simulink model "seesaw"  (Simulink 4.00)
settings: Solver=ode45  StartTime=0.0  StopTime=40  RelTol=1e-3
settings Model: Creator=tjanas  LastModifiedBy=tjanas  ExtModeAutoUpdateStatusClock=off  BooleanDataType=on

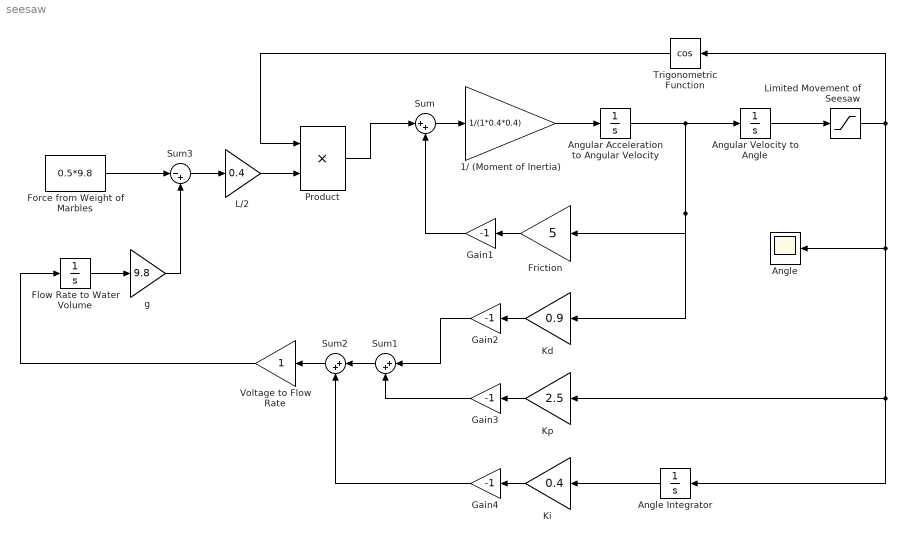
== system seesaw ==
  1/ (Moment of Inertia) : Gain  Gain=1/(1*0.4*0.4)  Multiplication=Element-wise(K.*u)  SaturateOnIntegerOverflow=on
  Angle : Scope
      settings: TimeRange=auto  YMin=-5  YMax=5  SaveToWorkspace=off  SaveName=ScopeData  LimitDataPoints=on  MaxDataPoints=5000
  Angle Integrator : Integrator  Orientation=left  ExternalReset=none  InitialConditionSource=internal  InitialCondition=1  LimitOutput=off  UpperSaturationLimit=inf  LowerSaturationLimit=-inf  ShowSaturationPort=off  ShowStatePort=off  AbsoluteTolerance=auto
  Angular Acceleration to Angular Velocity : Integrator  ExternalReset=none  InitialConditionSource=internal  InitialCondition=0  LimitOutput=off  UpperSaturationLimit=inf  LowerSaturationLimit=-inf  ShowSaturationPort=off  ShowStatePort=off  AbsoluteTolerance=auto
  Angular Velocity to Angle : Integrator  ExternalReset=none  InitialConditionSource=internal  InitialCondition=pi/12  LimitOutput=off  UpperSaturationLimit=inf  LowerSaturationLimit=-inf  ShowSaturationPort=off  ShowStatePort=off  AbsoluteTolerance=auto
  Flow Rate to Water Volume : Integrator  ExternalReset=none  InitialConditionSource=internal  InitialCondition=1  LimitOutput=off  UpperSaturationLimit=inf  LowerSaturationLimit=-inf  ShowSaturationPort=off  ShowStatePort=off  AbsoluteTolerance=auto
  Force from Weight of Marbles : Constant  Value=0.5*9.8
  Friction : Gain  Orientation=left  Gain=5  Multiplication=Element-wise(K.*u)  SaturateOnIntegerOverflow=on
  Gain{1..4} (4 alike) : Gain  Orientation=left  Gain=-1  Multiplication=Element-wise(K.*u)  SaturateOnIntegerOverflow=on
  Kd : Gain  Orientation=left  Gain=0.9  Multiplication=Element-wise(K.*u)  SaturateOnIntegerOverflow=on
  Ki : Gain  Orientation=left  Gain=0.4  Multiplication=Element-wise(K.*u)  SaturateOnIntegerOverflow=on
  Kp : Gain  Orientation=left  Gain=2.5  Multiplication=Element-wise(K.*u)  SaturateOnIntegerOverflow=on
  L/2 : Gain  Gain=0.4  Multiplication=Element-wise(K.*u)  SaturateOnIntegerOverflow=on
  Limited Movement of Seesaw : Saturate  UpperLimit=pi/12  LowerLimit=-pi/12  LinearizeAsGain=on
  Product : Product  Inputs=2  Multiplication=Element-wise(.*)  SaturateOnIntegerOverflow=on
  Sum : Sum  Inputs=|++  SaturateOnIntegerOverflow=on
  Sum1 : Sum  Orientation=left  Inputs=|++  SaturateOnIntegerOverflow=on
  Sum2 : Sum  Orientation=left  Inputs=|++  SaturateOnIntegerOverflow=on
  Sum3 : Sum  Inputs=|-+  SaturateOnIntegerOverflow=on
  Trigonometric Function : Trigonometry  Orientation=left  Operator=cos  OutputSignalType=auto
  Voltage to Flow Rate : Gain  Orientation=left  Gain=1  Multiplication=Element-wise(K.*u)  SaturateOnIntegerOverflow=on
  g : Gain  Gain=9.8  Multiplication=Element-wise(K.*u)  SaturateOnIntegerOverflow=on
  wires:
  Kd/1 -> Gain2/1
  Friction/1 -> Gain1/1
  Sum/1 -> 1/ (Moment of Inertia)/1
  1/ (Moment of Inertia)/1 -> Angular Acceleration to Angular Velocity/1
  Angular Acceleration to Angular Velocity/1 -> Angular Velocity to Angle/1, Friction/1, Kd/1
  Angular Velocity to Angle/1 -> Limited Movement of Seesaw/1
  Limited Movement of Seesaw/1 -> Trigonometric Function/1, Angle/1, Kp/1, Angle Integrator/1
  Gain1/1 -> Sum/2
  Kp/1 -> Gain3/1
  Ki/1 -> Gain4/1
  Angle Integrator/1 -> Ki/1
  Gain3/1 -> Sum1/2
  Gain2/1 -> Sum1/1
  Sum1/1 -> Sum2/1
  Gain4/1 -> Sum2/2
  Sum2/1 -> Voltage to Flow Rate/1
  Voltage to Flow Rate/1 -> Flow Rate to Water Volume/1
  Flow Rate to Water Volume/1 -> g/1
  g/1 -> Sum3/2
  Force from Weight of Marbles/1 -> Sum3/1
  Sum3/1 -> L/2/1
  L/2/1 -> Product/2
  Product/1 -> Sum/1
  Trigonometric Function/1 -> Product/1
